simulink model "sistema_pendolo"  (Simulink 7.5)
settings: Solver=ode45  StartTime=0.0  StopTime=10.0  RelTol=1e-3
values from neighbouring files (symbols this model uses):
  A = [0 1;-k/m -h/m]    [ctrl2.m]    (also in ctrl_obs_BUONO.m = [2 3;4 1]; es1.m = [2 3;4 1])
  C = [1 0]    [ctrl2.m]    (also in ctrl_obs_BUONO.m; es1.m)
  D = 0    [ctrl2.m]    (also in ctrl_obs_BUONO.m; es1.m)
  h = 0.5    [ctrl2.m]
  K = -place(A,B,aval_desiderati)    [ctrl2.m]    (also in ctrl_obs_BUONO.m = -place(A,B,aval_des); es1.m)
  L = -place(A',C',aval_obs_des)'    [ctrl_obs_BUONO.m]
  x0 = [1;0]    [ctrl2.m]    (also in ctrl_obs_BUONO.m = [1;1]; es1.m = [1;1])
  x0o = [0;0]    [ctrl_obs_BUONO.m]
undefined symbols (not defined in the file or in its folder): Bb, F1, F2, J, yeq1
libraries: simulink x1
settings Model: Creator=professore  LastModifiedBy=professore

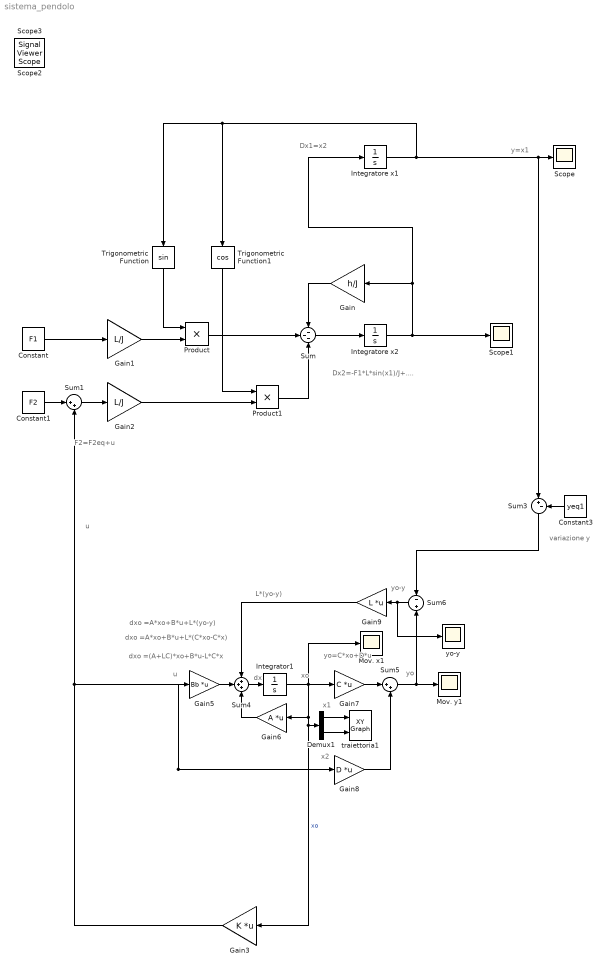
== system sistema_pendolo ==
  note: Dx1=x2
  note: Dx2=-F1*L*sin(x1)/J+....
  note: y=x1
  note: variazione y
  note: u
  note: F2=F2eq+u
  note: dxo =A*xo+B*u+L*(yo-y)
  note: yo=C*xo+D*u
  note: dx
  note: xo
  note: u
  note: x1
  note: x2
  note: yo
  note: yo-y
  note: L*(yo-y)
  note: dxo =A*xo+B*u+L*(C*xo-C*x)
  note: dxo =(A+LC)*xo+B*u-L*C*x
  Constant : Constant  Value=F1  OutDataType=fixdt(1, 16)  OutScaling=2^0
  Constant1 : Constant  Value=F2  OutDataType=fixdt(1, 16)  OutScaling=2^0
  Constant3 : Constant  Value=yeq1  OutDataType=fixdt(1, 16)  OutScaling=2^0
  Demux1 : Demux  Outputs=2
  Gain : Gain  Gain=h/J  ParameterDataType=fixdt(1, 16)  ParameterScaling=2^0  OutDataType=fixdt(1, 16)  OutScaling=2^0
  Gain1 : Gain  Gain=L/J  ParameterDataType=fixdt(1, 16)  ParameterScaling=2^0  OutDataType=fixdt(1, 16)  OutScaling=2^0
  Gain2 : Gain  Gain=L/J  ParameterDataType=fixdt(1, 16)  ParameterScaling=2^0  OutDataType=fixdt(1, 16)  OutScaling=2^0
  Gain3 : Gain  Gain=K  Multiplication=Matrix(K*u)  ParameterDataType=fixdt(1, 16)  ParameterScaling=2^0  OutDataType=fixdt(1, 16)  OutScaling=2^0
  Gain5 : Gain  Gain=Bb  Multiplication=Matrix(K*u)  ParameterDataType=fixdt(1, 16)  ParameterScaling=2^0  OutDataType=fixdt(1, 16)  OutScaling=2^0
  Gain6 : Gain  Gain=A  Multiplication=Matrix(K*u)  ParameterDataType=fixdt(1, 16)  ParameterScaling=2^0  OutDataType=fixdt(1, 16)  OutScaling=2^0
  Gain7 : Gain  Gain=C  Multiplication=Matrix(K*u)  ParameterDataType=fixdt(1, 16)  ParameterScaling=2^0  OutDataType=fixdt(1, 16)  OutScaling=2^0
  Gain8 : Gain  Gain=D  Multiplication=Matrix(K*u)  ParameterDataType=fixdt(1, 16)  ParameterScaling=2^0  OutDataType=fixdt(1, 16)  OutScaling=2^0
  Gain9 : Gain  Gain=L  Multiplication=Matrix(K*u)  ParameterDataType=fixdt(1, 16)  ParameterScaling=2^0  OutDataType=fixdt(1, 16)  OutScaling=2^0
  Integrator1 : Integrator  InitialCondition=x0o
  Integratore x1 : Integrator  InitialCondition=x0(1)
  Integratore x2 : Integrator  InitialCondition=x0(2)
  Mov. x1 : Scope
      settings: SaveName=ScopeData2
  Mov. y1 : Scope
      settings: SaveName=ScopeData3
  Product : Product  OutDataType=fixdt(1, 16)  OutScaling=2^0  RndMeth=Zero
  Product1 : Product  OutDataType=fixdt(1, 16)  OutScaling=2^0  RndMeth=Zero
  Scope : Scope
  Scope1 : Scope
  Sum : Sum  Inputs=---  OutDataType=fixdt(1, 16)  OutScaling=2^0
  Sum1 : Sum  Inputs=|++  OutDataType=fixdt(1, 16)  OutScaling=2^0
  Sum3 : Sum  Inputs=|+-  OutDataType=fixdt(1, 16)  OutScaling=2^0
  Sum4 : Sum  Inputs=+++  OutDataType=fixdt(1, 16)  OutScaling=2^0
  Sum5 : Sum  Inputs=|++  OutDataType=fixdt(1, 16)  OutScaling=2^0
  Sum6 : Sum  Inputs=-+  OutDataType=fixdt(1, 16)  OutScaling=2^0
  Trigonometric Function : Trigonometry
  Trigonometric Function1 : Trigonometry  Operator=cos
  traiettoria1 : simulink/Sinks/XY Graph  SystemSampleTime=-1  xmin=1  xmax=1.5  ymin=0  ymax=2  st=-1
  yo-y : Scope
      settings: SaveName=ScopeData4
  Scope2 : SignalViewerScope  IOType=viewer  RefreshTime=0.035000
  Scope3 : SignalViewerScope  IOType=viewer  RefreshTime=0.035000
  wires:
  Sum/1 -> Integratore x2/1
  Integratore x2/1 -> Integratore x1/1, Gain/1, Scope1/1
  Gain/1 -> Sum/1
  Gain1/1 -> Product/2
  Product/1 -> Sum/2
  Constant/1 -> Gain1/1
  Gain2/1 -> Product1/2
  Product1/1 -> Sum/3
  Trigonometric Function1/1 -> Product1/1
  Trigonometric Function/1 -> Product/1
  Integratore x1/1 -> Trigonometric Function/1, Trigonometric Function1/1, Scope/1, Sum3/1
  Constant1/1 -> Sum1/1
  Sum1/1 -> Gain2/1
  Constant3/1 -> Sum3/2
  Sum3/1 -> Sum6/1
  Gain3/1 -> Sum1/2, Gain5/1, Gain8/1
  Sum4/1 -> Integrator1/1
  Integrator1/1 -> Gain7/1, Gain6/1, Demux1/1, Gain3/1, Mov. x1/1  "xo"
  Gain7/1 -> Sum5/1
  Gain8/1 -> Sum5/2
  Sum5/1 -> Mov. y1/1, Sum6/2
  Demux1/1 -> traiettoria1/1
  Demux1/2 -> traiettoria1/2
  Sum6/1 -> Gain9/1, yo-y/1
  Gain9/1 -> Sum4/1
  Gain6/1 -> Sum4/3
  Gain5/1 -> Sum4/2
